simulink model "ilst_freqest_withEV"  (R2021a)
settings: Solver=ode45  StartTime=0.0  StopTime=2  RelTol=1e-3  EnableMultiTasking=on
undefined symbols (not defined in the file or in its folder): Ion, Lithium
libraries: spsCurrentMeasurementLib x25, spsVoltageMeasurementLib x19, spsSeriesRLCBranchLib x11, dspfdesign x6, spsGroundLib x6, powerlib_extras x4, dspsigops x3, spsPower3phInstantaneousLib x3, eeTotalHarmonicDistorsion x3, spsIGBTDiodeLib x2, spsUniversalBridgeLib x2, spsThreePhaseSourceLib x1
(part 2 of 2)

== system ilst_freqest_withEV/Control Algorithm/Subsystem6/Subsystem2 ==
  a : Inport
  Delay : Delay
  Delay1 : Delay
  Delay2 : Delay
  Differentiator Filter : dspfdesign/Differentiator Filter  DesignForMinimumOrder=on  FilterOrder=31  PassbandRipple=0.5  ScaleCoefficients=off  SimulateUsing=Interpreted execution  roundingMode=Floor  coeffsDataTypeStr=fixdt(1,16)
      settings: SourceProductBaseCode=DS
  Gain2 : Gain  Gain=200
  Gain6 : Gain  Gain=2
  Gain7 : Gain  Gain=10
  Product12 : Product
  Product13 : Product
  Sum12 : Sum  Inputs=-+
  Sum13 : Sum  Inputs=-+-+
  Sum14 : Sum  Inputs=+-
  Trigonometric Function : Trigonometry  Operator=acos  RemoveProtectionAgainstOutOfRangeInput=on
  Output : Outport
  wires:
  Delay1/1 -> Sum13/2, Sum12/1, Delay2/1
  Product13/1 -> Gain7/1
  Sum12/1 -> Gain6/1
  Gain7/1 -> Differentiator Filter/1
  Trigonometric Function/1 -> Gain2/1
  Delay/1 -> Sum13/3, Delay1/1
  Differentiator Filter/1 -> Product12/1, Trigonometric Function/1
  Product12/1 -> Sum14/2
  Delay2/1 -> Sum13/1
  Gain6/1 -> Product13/1, Product12/2
  Sum14/1 -> Product13/2
  Sum13/1 -> Sum14/1
  a/1 -> Sum13/4, Sum12/2, Delay/1
  Gain2/1 -> Output/1

== system ilst_freqest_withEV/PV Array/PV Module1/Subsystem ==
  note: Delta T
  note: Io
  Add4 : Sum  Inputs=+-
  Add5 : Sum
  Add6 : Sum
  Add7 : Sum  Inputs=+-
  Constant8 : Constant
  Divide2 : Product  Inputs=**
  Divide4 : Product  Inputs=*/
  Math Function1 : Math  SignedPower=on  SaturateOnIntegerOverflow=on
  Product4 : Product  RndMeth=Zero
  Product5 : Product  RndMeth=Zero
  Out1 : Outport
  wires:
  [Vt1] -> Divide2/2
  Divide4/1 -> Out1/1
  Add7/1 -> Divide4/2
  Divide2/1 -> Math Function1/1
  Constant8/1 -> Add7/2
  Math Function1/1 -> Add7/1
  Add6/1 -> Divide2/1
  Product5/1 -> Add6/1
  [Kv] -> Product5/2
  [Vocn1] -> Add6/2
  [Tn] -> Add4/2
  Add5/1 -> Divide4/1
  [Iscn1] -> Add5/1
  Product4/1 -> Add5/2
  [Ki] -> Product4/1
  Add4/1 -> Product5/1, Product4/2
  [T1] -> Add4/1

== system ilst_freqest_withEV/PV Array/PV Module1/Subsystem2 ==
  note: Ipv
  note: Delta T
  Add2 : Sum  Inputs=+-
  Add3 : Sum
  Divide1 : Product  Inputs=*/
  Product2 : Product  RndMeth=Zero
  Product3 : Product  RndMeth=Zero
  Out1 : Outport
  wires:
  [G1] -> Divide1/1
  [Gn] -> Divide1/2
  Divide1/1 -> Product3/2
  [Tn] -> Add2/2
  [T1] -> Add2/1
  Add2/1 -> Product2/2
  [Ki] -> Product2/1
  Product2/1 -> Add3/2
  [Ipvn1] -> Add3/1
  Add3/1 -> Product3/1
  Product3/1 -> Out1/1

== system ilst_freqest_withEV/PV Array/PV Module1/Vt ==
  note: Ns
  note: K
  note: q
  note: a
  note: T1
  Constant1 : Constant  Value=54
  Constant3 : Constant  Value=1.3806503e-23
  Constant6 : Constant  Value=1.60217646e-19
  Divide2 : Product  Inputs=*/
  Divide3 : Product  Inputs=/*
  Divide4 : Product  Inputs=***
  Vt : Outport
  wires:
  Divide3/1 -> Divide2/1
  Divide4/1 -> Divide3/1
  [T1] -> Divide2/2
  Constant6/1 -> Divide3/2
  Constant3/1 -> Divide4/3
  Constant1/1 -> Divide4/2
  [a] -> Divide4/1
  Divide2/1 -> Vt/1

== system ilst_freqest_withEV/Control Algorithm/Subsystem2/Subsystem1/Subsystem2 ==
  a : Inport
  Delay : Delay
  Delay1 : Delay
  Delay2 : Delay
  Differentiator Filter : dspfdesign/Differentiator Filter  DesignForMinimumOrder=on  FilterOrder=31  PassbandRipple=0.5  ScaleCoefficients=off  SimulateUsing=Interpreted execution  roundingMode=Floor  coeffsDataTypeStr=fixdt(1,16)
      settings: SourceProductBaseCode=DS
  Gain2 : Gain  Gain=200
  Gain6 : Gain  Gain=2
  Gain7 : Gain  Gain=10
  Product12 : Product
  Product13 : Product
  Sum12 : Sum  Inputs=-+
  Sum13 : Sum  Inputs=-+-+
  Sum14 : Sum  Inputs=+-
  Trigonometric Function : Trigonometry  Operator=acos  RemoveProtectionAgainstOutOfRangeInput=on
  Output : Outport
  wires:
  Delay1/1 -> Sum13/2, Sum12/1, Delay2/1
  Product13/1 -> Gain7/1
  Sum12/1 -> Gain6/1
  Gain7/1 -> Differentiator Filter/1
  Trigonometric Function/1 -> Gain2/1
  Delay/1 -> Sum13/3, Delay1/1
  Differentiator Filter/1 -> Product12/1, Trigonometric Function/1
  Product12/1 -> Sum14/2
  Delay2/1 -> Sum13/1
  Gain6/1 -> Product13/1, Product12/2
  Sum14/1 -> Product13/2
  Sum13/1 -> Sum14/1
  a/1 -> Sum13/4, Sum12/2, Delay/1
  Gain2/1 -> Output/1

== system ilst_freqest_withEV/Control Algorithm/Subsystem2/Subsystem2/Subsystem2 ==
  a : Inport
  Delay : Delay
  Delay1 : Delay
  Delay2 : Delay
  Differentiator Filter : dspfdesign/Differentiator Filter  DesignForMinimumOrder=on  FilterOrder=31  PassbandRipple=0.5  ScaleCoefficients=off  SimulateUsing=Interpreted execution  roundingMode=Floor  coeffsDataTypeStr=fixdt(1,16)
      settings: SourceProductBaseCode=DS
  Gain2 : Gain  Gain=200
  Gain6 : Gain  Gain=2
  Gain7 : Gain  Gain=10
  Product12 : Product
  Product13 : Product
  Sum12 : Sum  Inputs=-+
  Sum13 : Sum  Inputs=-+-+
  Sum14 : Sum  Inputs=+-
  Trigonometric Function : Trigonometry  Operator=acos  RemoveProtectionAgainstOutOfRangeInput=on
  Output : Outport
  wires:
  Delay1/1 -> Sum13/2, Sum12/1, Delay2/1
  Product13/1 -> Gain7/1
  Sum12/1 -> Gain6/1
  Gain7/1 -> Differentiator Filter/1
  Trigonometric Function/1 -> Gain2/1
  Delay/1 -> Sum13/3, Delay1/1
  Differentiator Filter/1 -> Product12/1, Trigonometric Function/1
  Product12/1 -> Sum14/2
  Delay2/1 -> Sum13/1
  Gain6/1 -> Product13/1, Product12/2
  Sum14/1 -> Product13/2
  Sum13/1 -> Sum14/1
  a/1 -> Sum13/4, Sum12/2, Delay/1
  Gain2/1 -> Output/1

== system ilst_freqest_withEV/Control Algorithm/Subsystem2/Subsystem3/Subsystem2 ==
  a : Inport
  Delay : Delay
  Delay1 : Delay
  Delay2 : Delay
  Differentiator Filter : dspfdesign/Differentiator Filter  DesignForMinimumOrder=on  FilterOrder=31  PassbandRipple=0.5  ScaleCoefficients=off  SimulateUsing=Interpreted execution  roundingMode=Floor  coeffsDataTypeStr=fixdt(1,16)
      settings: SourceProductBaseCode=DS
  Gain2 : Gain  Gain=200
  Gain6 : Gain  Gain=2
  Gain7 : Gain  Gain=10
  Product12 : Product
  Product13 : Product
  Sum12 : Sum  Inputs=-+
  Sum13 : Sum  Inputs=-+-+
  Sum14 : Sum  Inputs=+-
  Trigonometric Function : Trigonometry  Operator=acos  RemoveProtectionAgainstOutOfRangeInput=on
  Output : Outport
  wires:
  Delay1/1 -> Sum13/2, Sum12/1, Delay2/1
  Product13/1 -> Gain7/1
  Sum12/1 -> Gain6/1
  Gain7/1 -> Differentiator Filter/1
  Trigonometric Function/1 -> Gain2/1
  Delay/1 -> Sum13/3, Delay1/1
  Differentiator Filter/1 -> Product12/1, Trigonometric Function/1
  Product12/1 -> Sum14/2
  Delay2/1 -> Sum13/1
  Gain6/1 -> Product13/1, Product12/2
  Sum14/1 -> Product13/2
  Sum13/1 -> Sum14/1
  a/1 -> Sum13/4, Sum12/2, Delay/1
  Gain2/1 -> Output/1

== matlab function ilst_freqest_withEV/MPPT ==
  settings: updateMethod=DISCRETE  sampleTime=1e-4
  data: tv input; Ipvin input; Vpvin input; Ipvin1 input; Vpvin1 input; Vdcref output; Vdcrefold input
function Vdcref = fcn(tv,Ipvin,Vpvin,Ipvin1,Vpvin1,Vdcrefold)
%#codegen
delVdc=0.2;
a=10;
delVpv=Vpvin-Vpvin1;
delIpv=Ipvin-Ipvin1;
if(tv>=0.6)
if(delVpv==0)
    if(delIpv==0)
        Vdcrefnew=Vdcrefold;
    else
        if(delIpv>0)
            Vdcrefnew=Vdcrefold-(delIpv/delVpv)*a;
    else
        Vdcrefnew=Vdcrefold+(delIpv/delVpv)*a;
        end
    end
    else
        if(delIpv/delVpv==-Ipvin/Vpvin)
            Vdcrefnew=Vdcrefold;
        else
            if(delIpv/delVpv>-Ipvin/Vpvin)
                Vdcrefnew=Vdcrefold-(delIpv/delVpv)*a;
            else
                Vdcrefnew=Vdcrefold+(delIpv/delVpv)*a;
            end
        end
end
Vdcref=Vdcrefnew;
else
Vdcref=810;
end


%Vdcref=658;
